simulink model "Lab_3_Receiver_Daniel_J_Lopes"  (R2021b)
settings: Solver=FixedStepDiscrete  StartTime=0.0  StopTime=inf  RelTol=1e-3
PreLoadFcn:
  | platform = sdruExampleFindRadio;
  | frsRxParams = getParamsSdruFRSGMRSRxDemo(platform);
  | clear platform
PostLoadFcn:
  | sdruExampleSetAvailableRadio;
InitFcn:
  | platform = get_param([gcs '/SDRu Receiver'], 'Platform');
  | frsRxParams = getParamsSdruFRSGMRSRxDemo(platform);
  | switch platform
  |   case 'X300'
  |     set_param([gcs,'/SDRu Receiver'], 'masterClkRateX300','200e6');
  |   case 'X310'
  |     set_param([gcs,'/SDRu Receiver'], 'masterClkRateX310','200e6');
  |   case 'N300'
  |     set_param([gcs,'/SDRu Receiver'], 'masterClkRateN300','153.6e6');
  |   case 'N310'
  |     set_param([gcs,'/SDRu Receiver'], 'masterClkRateN310','153.6e6');
  |   case 'N320/N321'
  |     set_param([gcs,'/SDRu Receiver'], 'masterClkRateN320','200e6');
  | end
  | clear platform
undefined symbols (not defined in the file): fdesignblkfcn, frsRxCTCSSDecodeBlockLength, frsRxCTCSSToneFrequencies, frsRxGoertzelCoefficients, Fs, gcbh, ip, usb
libraries: plutoradiolib x1, commrfcorlib x1, dspsnks4 x1, dspmlti4 x1, commanabbnd3 x1, sdrublksprivate x1, sdrrlib x1, commsdrhw_v2 x1, simulink x1
Description:
  | This model uses Simulink(R) to receive a Family Radio Service (FRS) signal from Universal Software Radio Peripheral (USRP) hardware.
settings Model: Creator=The MathWorks, Inc.  LastModifiedBy=Daniel
settings SolverCC: AlgebraicLoopSolver=TrustRegion
settings DataIOCC: SaveFormat=Array  SaveOutput=off  SignalLogging=off  DSMLogging=off  SaveTime=off  ReturnWorkspaceOutputs=off
settings OptimizationCC: ExpressionDepthLimit=2147483647  LifeSpan=inf  SimCompilerOptimization=on
settings DebuggingCC: UnderspecifiedInitializationDetection=Classic  MergeDetectMultiDrivingBlocksExec=none  SolverPrmCheckMsg=warning  InheritedTsInSrcMsg=none  MultiTaskCondExecSysMsg=none  ParameterPrecisionLossMsg=none  FcnCallInpInsideContextMsg=warning  AllowSymbolicDim=off  StateNameClashWarn=warning  SFUnexpectedBacktrackingDiag=warning  SFNoUnconditionalDefaultTransitionDiag=warning  SFExecutionAtInitializationDiag=none  SFMachineParentedDataDiag=warning  ArithmeticOperatorsInVariantConditions=warning
settings HardwareCC: ProdBitPerPointer=32  ProdBitPerSizeT=32  ProdBitPerPtrDiffT=32  ProdLargestAtomicFloat=None  ProdIntDivRoundTo=Undefined  ProdEndianess=Unspecified  ProdWordSize=32  ProdHWDeviceType=32-bit Generic  TargetBitPerPointer=64  TargetBitPerSizeT=64  TargetBitPerPtrDiffT=64  TargetLongLongMode=on  TargetIntDivRoundTo=Zero  TargetEndianess=LittleEndian  TargetWordSize=64  TargetHWDeviceType=Generic->MATLAB Host Computer  ProdEqTarget=off
settings ModelReferenceCC: PropagateSignalLabelsOutOfModel=off
settings SFSimCC: SimIntegrity=off  SimUseLocalCustomCode=off  CustomCodeUndefinedFunction=UseInterfaceOnly
settings RTWCC: RTWUseLocalCustomCode=off
settings RTWCC: CustomSourceCode=|
  | #include <stdio.h>
  | #include <stdlib.h>
settings CodeAppCC: StateflowObjectComments=on
settings GRTTargetCC: TargetLangStandard=C89/C90 (ANSI)  CombineOutputUpdateFcns=off  GRTInterface=on
settings ConfigComp: CovMetricSettings=dw  CovSaveCumulativeToWorkspaceVar=on  CovSaveSingleToWorkspaceVar=on  CovExternalEMLEnable=off  CovSFcnEnable=off

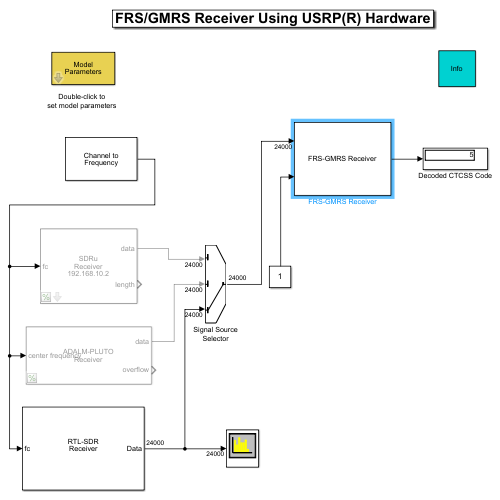
[thumbnail: Simulink's stored preview of the top-level diagram]
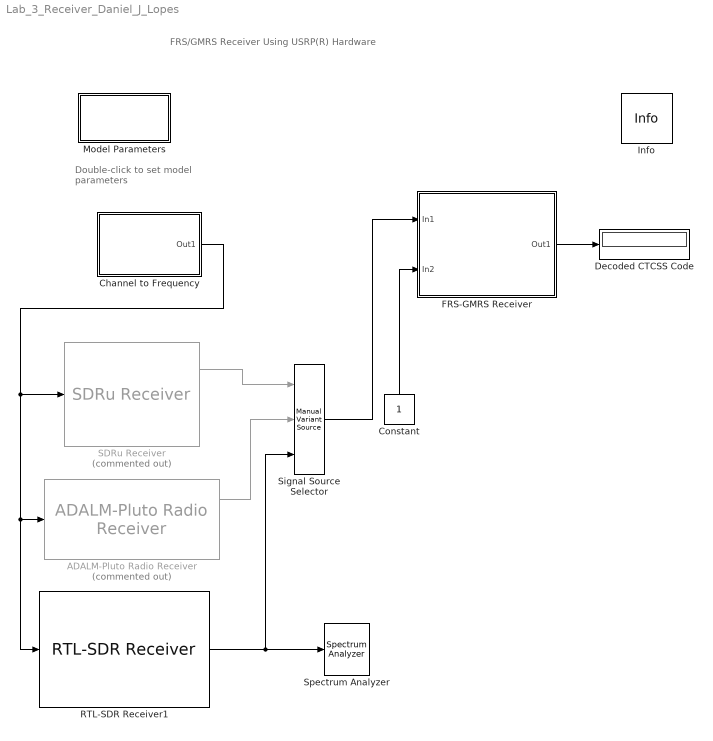
== system Lab_3_Receiver_Daniel_J_Lopes ==
  note: FRS/GMRS Receiver Using USRP(R) Hardware
  note: Double-click to
      | set model parameters
  ADALM-Pluto Radio Receiver : plutoradiolib/ADALM-Pluto Radio Receiver  Commented=on  RadioID=usb:0  uri=ip:10.0.0.200  CenterFrequencySource=Input Port  CenterFrequency=2.4e9  GainSource=AGC Slow Attack  GainSourceBlock=AGC Slow Attack  Gain=10  ChannelMapping=1  BasebandSampleRate=1e6  OutputDataType=single  SamplesPerFrame=4000  OverflowOutputPort=on  EnableBurstMode=off  NumFramesInBurst=1  ShowAdvancedProperties=off  UseCustomFilter=off  filtPathRates=[737280000 11520000 3840000 1920000 960000 240000]  filtCoefficients=[-192 82 85 -215 228 -102 -110 290 -318 145 160 -426 471 -215 -238 633 -697 318 349 -923 1009 -457 -498 1309 -1423 640 693 -1812 1959 -876 -945 2458 -2647 1180 1268 -3290 3534 -1572 -1688 4375 -4698 2091 2247 -5836 6284 -2807 -3031 7918 -8588 3870 4225 -11182 12324 -5662 -6330 17255 -19735 9507 11312 -33568 43355 -25227 -42139 305542 305542 -42139 -25227 43355 -33568 11312 9507 -19735 17255 -6330 -5662 12324 -11182 4225 3870 -8588 7918 -3031 -2807 6284 -5836 2247 2091 -4698 4375 -1688 -1572 3534 -3290 1268 1180 -2647 2458 -945 -876 1959 -1812 693 640 -1423 1309 -498 -457 1009 -923 349 318 -697 633 -238 -215 471 -426 160 145 -318 290 -110 -102 228 -215 85 82 -192]  filtCoefficientSize=128  filtDecimInterpFactor=4  filtGain=-12  filtRFBandwidth=18000000  filterConfigStruct=struct()  EnableQuadratureCorrection=on  EnableRFDCCorrection=on  EnableBasebandDCCorrection=on  FrequencyCorrection=0  OverrideSampleTime=off  SampleTime=0.02  DataTimeout=Inf  ENSMPinControlMode=None  BISTLoopbackMode=Disabled  BISTToneInject=Disabled  BISTSignalGen=PRBS  BISTToneFreq=Fs/32  BISTToneLevel=0
      settings: SourceProductBaseCode=PLUTO
  Channel to Frequency : Subsystem
      mask Display: disp('Channel to\nFrequency');
  Constant : Constant
  Decoded CTCSS Code : Display
  FRS-GMRS Receiver : Subsystem
      mask Display: disp('FRS-GMRS Receiver');
  Info : sdrublksprivate/Info  SystemSampleTime=-1  VariantActivationTime=update diagram  Latency=0  AutoFrameSizeCalculation=off
      settings: SourceProductBaseCode=USRP
  Model Parameters : Subsystem  mask(Model Parameters){channel=1, code=5, decodeThresh=0.1}
      mask prompts: channel "Channel (1 to 14):"; code "CTCSS Code (0 to 38):"; decodeThresh "Average signal threshold for squelch:"
      mask help: Specifies model parameters for a simulation run.
      mask init:
      | usrpFRSGMRS_mask(gcbh, 'init', 'rec', channel, code, decodeThresh);
      mask Help: eval('usrpdemohelp');
      mask Display: disp('Model\nParameters');
  RTL-SDR Receiver1 : sdrrlib/RTL-SDR Receiver  IPAddress=0  CenterFrequencySource=Input port  CenterFrequency=102.5e6  GainSource=AGC  Gain=0  ADCRate=240e3  FrequencyCorrection=0  LostSamplesOutputPort=off  LatencyOutputPort=off  OutputDataType=double  FrameLength=24000  EnableBurstMode=off  NumFramesInBurst=20  sobjType=sdrr.internal.SDRRTLReceiverSL  dataUDPPort=-1  ctrlUDPPort=-1  subDeviceList=nosubdev  sdrBlockType=SDRBlockTypeSLT.SDRRxBlock  requester=UNUSED_BY_SFCN  sdrExecutionMode=SDRExecutionModeSLT.ExecModeHW  BypassUserLogic=off  DecimatorSelect=DDC decimator  SourceSelect=RF data  SineAmplitude=16000  EnableInternalClock=off  BypassIQBalance=off  IFBandwidth=40e6  ADCRateSource=Dialog  IntermediateFrequency=0  DecimationFactorSource=Dialog  DecimationFactor=512  RFFrequencyIsTunable=logical(1)  SampleTime=(24000)/(240e3)  IFBandwidthSource=Dialog  SineFrequency=30000  BypassDCBlockingFilter=off  IntermediateFrequencySource=Dialog  IQBalanceCoefficients=64  SkipAllHardwareResetAndInitialization=off  EnableIQCalibrationTable=on  CacheIQCalibrationTable=off  EnableOffsetTuning=off  EnableRTLAGC=off  EnableTestMode=off  EnableTunerAGC=on  FrequencyCorrectionSource=Dialog  NumMLBuffers=128  NumUSBBuffers=16  RTLCrystalFrequency=28800000  TunerCrystalFrequency=28800000
      settings: SourceProductBaseCode=RTLSDR
  SDRu Receiver : commsdrhw_v2/SDRu Receiver  Commented=on  rxtx=rx  initializeIPAddress=0  devMap=10  USRP2_IP=192.168.10.2  USRP_IP_X300=192.168.10.2  USRP_IP_X310=192.168.10.2  USRP_IP_N300=192.168.10.2  USRP_IP_N310=192.168.10.2  USRP_IP_N320=192.168.10.2  USRP_serialNumB200=30FD838  USRP_serialNumB210=3136D5F  platform=N200/N210/USRP2  prevPlatform=N200/N210/USRP2  lastIPAddressPopup=192.168.10.2  USRP_ID=192.168.10.2  LastIPAddress=192.168.10.2  IsTwinRXDaughterboard=off  EnableTwinRXPhaseSync=off  losrc=0  ChannelMapping=1  centerFrequencySrc=Input port  centerFrequency=2.45e9  loOffsetSrc=Dialog  loOffset=0  gainSrc=Dialog  gain=frsRxParams.RadioGain  PPSSource=GPSDO  EnableGPSLock=off  EnsureSyncGPSTime=off  clockSource=GPSDO  EnableRefLock=off  masterClkRateParam=100e6  masterClkRateB200=frsRxParams.RadioMasterClockRate  masterClkRateB210=frsRxParams.RadioMasterClockRate  masterClkRateX300=200e6  masterClkRateX310=200e6  masterClkRateN300=153.6e6  masterClkRateN310=153.6e6  masterClkRateN320=200e6  masterClkRate=100e6  masterClkRateTwinRX=200e6  decimInterpSrc=Dialog  decimInterpPort=512  lastDecimSource=Dialog  decimInterp=frsRxParams.RadioDecimationFactor  USRP2_IP_NUM=[49 57 50 46 49 54 56 46 49 48 46 50]  sampleRate=200000  sampleTime=500/100000000  TransportDataType=int16  overrunUnderrunPort=off  outputDatatype=single  frameLength=frsRxParams.RadioFrameLength  HOST_DATA_PORT=30000  HOST_CONTROL_PORT=30002  USRP2_DATA_PORT=32769  USRP2_CONTROL_PORT=32768  bufferMode=Continuous streaming  EnableBurstMode=off  NumFramesInBurst=100
      settings: SourceProductBaseCode=USRP
  Signal Source Selector : simulink/Signal Routing/Manual Variant Source  NumChoices=3  LabelModeActiveChoice=V_3
  Spectrum Analyzer : SpectrumAnalyzer
  wires:
  FRS-GMRS Receiver/1(Out1) -> Decoded CTCSS Code/1
  Channel to Frequency/1(Out1) -> RTL-SDR Receiver1/1, ADALM-Pluto Radio Receiver/1, SDRu Receiver/1
  SDRu Receiver/1 -> Signal Source Selector/1
  ADALM-Pluto Radio Receiver/1 -> Signal Source Selector/2
  RTL-SDR Receiver1/1 -> Spectrum Analyzer/1, Signal Source Selector/3
  Signal Source Selector/1 -> FRS-GMRS Receiver/1(In1)
  Constant/1 -> FRS-GMRS Receiver/2(In2)

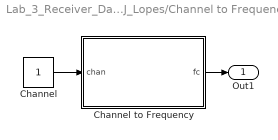
== system Lab_3_Receiver_Daniel_J_Lopes/Channel to Frequency ==
  Channel : Constant  VectorParams1D=off  OutDataTypeStr=uint16  SampleTime=-1  FramePeriod=-1
  Channel to Frequency : MATLAB Function  TreatAsAtomicUnit=on
  Out1 : Outport  VectorParamsAs1DForOutWhenUnconnected=off
  wires:
  Channel/1 -> Channel to Frequency/1(chan)
  Channel to Frequency/1(fc) -> Out1/1

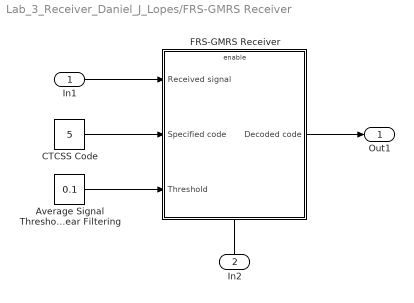
== system Lab_3_Receiver_Daniel_J_Lopes/FRS-GMRS Receiver ==
  In1 : Inport
  In2 : Inport  Port=2
  Average Signal Threshold for Nonlinear Filtering : Constant  Value=0.1  VectorParams1D=off  OutDataTypeStr=single  FramePeriod=-1
  CTCSS Code : Constant  Value=5  OutDataTypeStr=uint8
  FRS-GMRS Receiver : Subsystem  TreatAsAtomicUnit=on
  Out1 : Outport  VectorParamsAs1DForOutWhenUnconnected=off
  wires:
  CTCSS Code/1 -> FRS-GMRS Receiver/2(Specified code)
  Average Signal Threshold for Nonlinear Filtering/1 -> FRS-GMRS Receiver/3(Threshold)
  In1/1 -> FRS-GMRS Receiver/1(Received signal)
  FRS-GMRS Receiver/1(Decoded code) -> Out1/1
  In2/1 -> FRS-GMRS Receiver/Enable

== system Lab_3_Receiver_Daniel_J_Lopes/Model Parameters ==
  note: This subsystem is empty.
      | It is used for setting parameter values (in the mask).

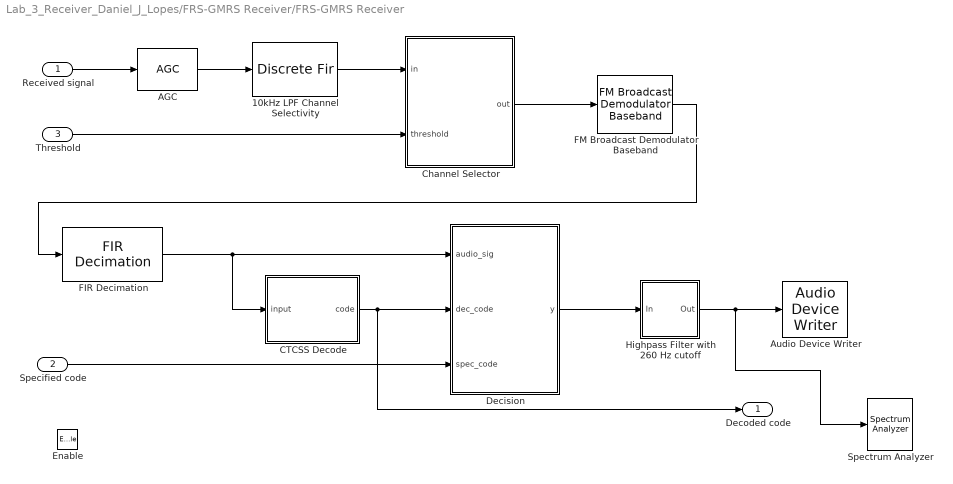
== system Lab_3_Receiver_Daniel_J_Lopes/FRS-GMRS Receiver/FRS-GMRS Receiver ==
  Received signal : Inport
  Specified code : Inport  Port=2
  Threshold : Inport  Port=3
  Enable : EnablePort
  10kHz LPF Channel Selectivity : DiscreteFir  Coefficients=frsRxParams.ChannelFilterNumerator  InputProcessing=Columns as channels (frame based)  OutDataTypeStr=fixdt(1,16,0)
      settings: LockScale=on
  AGC : commrfcorlib/AGC  LegacyMode=off  DetectorMethod=Rectifier  LoopMethod=Linear  UpdatePeriod=1  StepSize=1  AdaptationStepSize=0.01  DesiredOutputPower=1  AveragingLength=100  MaximumGain=1e6  MaxPowerGain=60  GainOutputPort=off  InputPowerOutputPort=off  SimulateUsing=Code generation
  Audio Device Writer : dspsnks4/Audio Device Writer  Driver=DirectSound  Device=LC24RG50 (NVIDIA High Definition Audio)  InheritSampleRate=on  SampleRate=48000  BitDepth=16-bit integer  BufferSize=4096  NumBuffers=10  DefaultOutputChannelMapping=on  OutputChannelMapping=1:2  OutputNumUnderrunSamples=off  DriverIdx=1  DeviceWarnFlag=''
  CTCSS Decode : MATLAB Function  TreatAsAtomicUnit=on
  Channel Selector : MATLAB Function  TreatAsAtomicUnit=on
  Decision : MATLAB Function  TreatAsAtomicUnit=on
  FIR Decimation : dspmlti4/FIR Decimation  FilterSource=Auto  h=frsRxParams.DecimationNumerator  D=30  filtStruct=Direct form  FilterObject=FDECIM  InputProcessing=Columns as channels (frame based)  framing=Enforce single-rate processing  inputOffset=0  outputBufInitCond=0  roundingMode=Floor  overflowMode=off  firstCoeffDataTypeStr=Inherit: Same word length as input  firstCoeffMin=[]  firstCoeffMax=[]  firstCoeffLastDataTypeStr=Inherit: Same word length as input  outputDataTypeStr=Inherit: Same as accumulator  outputMin=[]  outputMax=[]  outputLastDataTypeStr=Inherit: Same as accumulator
  FM Broadcast Demodulator Baseband : commanabbnd3/FM Broadcast Demodulator Baseband  SampleRate=288e3  FrequencyDeviation=2500  FilterTimeConstant=75e-6  AudioSampleRate=288e3  PlaySound=off  BufferSize=4096  Stereo=off  RBDS=off  RBDSSamplesPerSymbol=10  RBDSCostasLoop=off  SimulateUsing=Interpreted execution
      settings: SourceProductBaseCode=CM
  Highpass Filter with 260 Hz cutoff : Subsystem  DialogController=fdesignblkfcn  InitFcn=fdesignblkfcn(gcbh, {'InitFcn'});  mask(Highpass Filter){}
      mask help: Design a highpass filter
      settings: CopyFcn=fdesignblkfcn(gcbh, {'CopyFcn'});
      mask Help: helpview(mapfilelocation('dsp'), 'dsphighpassfilter');
      mask Display: disp('Highpass')
  Spectrum Analyzer : SpectrumAnalyzer
  Decoded code : Outport  VectorParamsAs1DForOutWhenUnconnected=off
  wires:
  Received signal/1 -> AGC/1
  10kHz LPF Channel Selectivity/1 -> Channel Selector/1(in)
  AGC/1 -> 10kHz LPF Channel Selectivity/1
  Decision/1(y) -> Highpass Filter with 260 Hz cutoff/1(In)
  FIR Decimation/1 -> Decision/1(audio_sig), CTCSS Decode/1(input)
  Specified code/1 -> Decision/3(spec_code)
  Threshold/1 -> Channel Selector/2(threshold)
  CTCSS Decode/1(code) -> Decision/2(dec_code), Decoded code/1
  Channel Selector/1(out) -> FM Broadcast Demodulator Baseband/1
  FM Broadcast Demodulator Baseband/1 -> FIR Decimation/1
  Highpass Filter with 260 Hz cutoff/1(Out) -> Spectrum Analyzer/1, Audio Device Writer/1

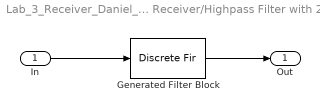
== system Lab_3_Receiver_Daniel_J_Lopes/FRS-GMRS Receiver/FRS-GMRS Receiver/Highpass Filter with 260 Hz cutoff ==
  In : Inport
  Generated Filter Block : DiscreteFir  Tag=BlockMethodSubSystem  Coefficients=[-6.7061602858709636e-05 0.02315973133211649 -0.0019581084510045996 -0.0021236298041915065 -0.0023022277358131097 -0.0025599768128848066 -0.0028226592821177661 -0.0030731159919254996 -0.0032631866911224205 -0.0033525027873635375 -0.0033110925699644336 -0.0031138934572151286 -0.0027428261193899036 -0.0022006879446808451 -0.0014938732079750462 -0.00064932035493273522 0.00029711032998214123 0.0012967030335343283 0.0022942825383397251 0.0032255484079617295 0.0040300085817981755 0.0046439332728520364 0.0050154276835890623 0.0050997277778646738 0.0048696503592197838 0.0043124955901376293 0.003439067405142879 0.0022763146230193542 0.00087632604777342397 -0.00069412704606115652 -0.0023485014983496218 -0.0039913718535405868 -0.0055167223400405417 -0.0068210699814491337 -0.0078016630505272581 -0.0083713052593811163 -0.0084567493812427331 -0.0080113702580126758 -0.0070134156788826847 -0.0054761667431133497 -0.0034424053618224717 -0.0009926264256152255 0.001764430988736114 0.0046885025780096529 0.0076187204304470346 0.010375174033707657 0.012773021641220957 0.01462418559028229 0.015754835422537718 0.016007639739238091 0.015255703780429553 0.01340778178166049 0.010416806044496173 0.0062808572184119994 0.0010521634131988511 -0.0051707337099740989 -0.012239496836442359 -0.019960370571649063 -0.02810829437200273 -0.036425485744674579 -0.044637995084667308 -0.052470002238885871 -0.059648362537931272 -0.065907928939195726 -0.071055009001286237 -0.07484982685839317 -0.077190657100754179 0.92194882982973714 -0.077190657100754179 -0.07484982685839317 -0.071055009001286237 -0.065907928939195726 -0.059648362537931272 -0.052470002238885871 -0.044637995084667308 -0.036425485744674579 -0.02810829437200273 -0.019960370571649063 -0.012239496836442359 -0.0051707337099740989 0.0010521634131988511 0.0062808572184119994 0.010416806044496173 0.01340778178166049 0.015255703780429553 0.016007639739238091 0.015754835422537718 0.01462418559028229 0.012773021641220957 0.010375174033707657 0.0076187204304470346 0.0046885025780096529 0.001764430988736114 -0.0009926264256152255 -0.0034424053618224717 -0.0054761667431133497 -0.0070134156788826847 -0.0080113702580126758 -0.0084567493812427331 -0.0083713052593811163 -0.0078016630505272581 -0.0068210699814491337 -0.0055167223400405417 -0.0039913718535405868 -0.0023485014983496218 -0.00069412704606115652 0.00087632604777342397 0.0022763146230193542 0.003439067405142879 0.0043124955901376293 0.0048696503592197838 0.0050997277778646738 0.0050154276835890623 0.0046439332728520364 0.0040300085817981755 0.0032255484079617295 0.0022942825383397251 0.0012967030335343283 0.00029711032998214123 -0.00064932035493273522 -0.0014938732079750462 -0.0022006879446808451 -0.0027428261193899036 -0.0031138934572151286 -0.0033110925699644336 -0.0033525027873635375 -0.0032631866911224205 -0.0030731159919254996 -0.0028226592821177661 -0.0025599768128848066 -0.0023022277358131097 -0.0021236298041915065 -0.0019581084510045996 0.02315973133211649 -6.7061602858709636e-05]  InputProcessing=Columns as channels (frame based)
  Out : Outport  VectorParamsAs1DForOutWhenUnconnected=off
  wires:
  Generated Filter Block/1 -> Out/1
  In/1 -> Generated Filter Block/1

== matlab function Lab_3_Receiver_Daniel_J_Lopes/FRS-GMRS Receiver/FRS-GMRS Receiver/Channel Selector ==
  data: in input; out output size=[24000, 1]; threshold input
function out = channelSelector(in, threshold)
%#codegen
% Compute the average power of the input signal, if
% it is greater than a threshold, let the signal go through, otherwise,
% mute. 

len = length(in); 
power = sum(abs(in)) / len;

if (power >= threshold)
    out = in;
else 
    %out = single(zeros(len,1));
    out = double(zeros(len,1));
end

== matlab function Lab_3_Receiver_Daniel_J_Lopes/FRS-GMRS Receiver/FRS-GMRS Receiver/Decision ==
  data: audio_sig input; y output size=[800, 1]; dec_code input; spec_code input
function y  = decision(audio_sig, dec_code, spec_code)
%#codegen

% If the decoded code equals to pre-specified code, or the pre-specified
% code is 0 (no CTCSS), the audio signal goes through, otherwise, output
% zero.

if ((dec_code == spec_code) || (spec_code == 0))
    y = audio_sig;
else
    %y = single(zeros(length(audio_sig),1));
    y = double(zeros(length(audio_sig),1));
end

== matlab function Lab_3_Receiver_Daniel_J_Lopes/Channel to Frequency/Channel to Frequency ==
  data: chan input uint16; fc output double
function fc = ChanToFreq(chan)
%#codegen
% Map integer channel number to FRS/GMRS center frequencies

fc = convertChan2FreqFRSGMRSDemo(chan);

== matlab function Lab_3_Receiver_Daniel_J_Lopes/FRS-GMRS Receiver/FRS-GMRS Receiver/CTCSS Decode ==
  data: input input; code output int8; frsRxCTCSSToneFrequencies parameter; frsRxGoertzelCoefficients parameter; frsRxCTCSSDecodeBlockLength parameter
function code  = CTCSS_Decode(input, frsRxCTCSSToneFrequencies, ...
    frsRxGoertzelCoefficients, frsRxCTCSSDecodeBlockLength)
%#codegen
% CTCSS decoder for use in a tone squelch system.
%
% Requires identification of one of a set of tones in the audio stream.
% Input is a frame of audio samples at a sample rate of (close to) 8kHz.
%
% Each time the function is called when a frame of samples comes in. It
% changes the state of the function, s(n), s(n-1), s(n-2). When a block of
% samples passes through (block size specified by frs_decodeBlockSize ),
% the power at each frequency is computed by Goertzel algorithm and the
% state is cleared to zero, preparing for the next block. The block size
% could be much larger than the frame size. 
%
% Below is the frequency table for private codes. 
% 
% PL   Hz     PL   Hz      PL   Hz
% --  ----    --  -----    --  -----
%  1  67.0    12  100.0    32  203.5
%  2  71.9    13  103.5    33  210.7
%  3  74.4    14  107.2    34  218.1
%  4  77.0    15  110.9    35  225.7
%  5  79.7    16  114.8    36  233.6
%  6  82.5    17  118.8    37  241.8
%  7  85.4    18  123.0    38  250.3
%  8  88.5    19  127.3
%  9  91.5    20  131.8
% 10  94.8    21  136.5
% 11  97.4    22  141.3
%             23  146.2
%             24  151.4
%             25  156.7
%             26  162.2
%             27  167.9
%             28  173.8
%             29  179.9
%             30  186.2
%             31  192.8

nTones = length(frsRxCTCSSToneFrequencies);

persistent  s_d1 s_d2 s maxPowerIdx nProcessed

if isempty(s_d1)
    s_d1 = coder.nullcopy(single(zeros(nTones,1)));% s_d1 = s(n-1)
    s_d2 = coder.nullcopy(single(zeros(nTones,1)));% s_d2 = s(n-2)
    s = coder.nullcopy(single(zeros(nTones,1))); % s = s(n)
    nProcessed = 0;
    maxPowerIdx = 0; 
end

frameSize = length(input);

% The number of sample needs to be processed
%nSampleProc = min(frameSize, frsRxCTCSSDecodeBlockLength - nProcessed);
nSampleProc = min(frameSize, 24e3 - nProcessed);

for i = 1:nSampleProc
	inputVec = repmat(input(i), nTones,1);
	s  = inputVec + frsRxGoertzelCoefficients .* s_d1 - s_d2; % s(n) = x(n) + 2cos(2*pi*w)s(n-1) - s(n-2)
	s_d2 = s_d1;
	s_d1 = s;
end

nProcessed  = nProcessed + nSampleProc;

% if a block is done
if (nProcessed == frsRxCTCSSDecodeBlockLength)
	
	power = s_d2.^2 + s_d1.^2 - frsRxGoertzelCoefficients .* s_d2 .* s_d1;

    if (any(power ~= 0))
        [~, maxPowerIdx] = max(power);
    end

    % clear the state
	s_d1 = single(zeros(nTones,1));
	s_d2 = single(zeros(nTones,1));
	
    % next block starts, process the remaining samples in the current frame
	for i = nSampleProc + 1 : frameSize
		inputVec = repmat(input(i), nTones,1);
		s  = inputVec + frsRxGoertzelCoefficients .* s_d1 - s_d2;
		s_d2 = s_d1;
		s_d1 = s;
	end
	nProcessed = frameSize - nSampleProc;

end

code = int8(maxPowerIdx);
